simulink model "uni_model_v3"  (R2017b)
settings: Solver=FixedStepDiscrete  StartTime=0.0  StopTime=time  FixedStep=dt  RelTol=1e-3
values from neighbouring files (symbols this model uses):
  dt = 0.1    [extendedKalmanFilter.m]    (also in matlab.mat; runV3.m; rungen.m; runpathfollower.m)
  i0 = 0    [matlab.mat]    (also in runV3.m = [0 0]')
  xi0 = [0 0 0 0 0 0 0 0]    [matlab.mat]    (also in runV3.m = [0 0 0 0 0 0 0 0]'; runpathfollower.m = [xi,yi,0,0,0,0,theta_mi,0]'; runpathplanner.m = [xi,yi,0,0,0,0,theta_mi,0]')
undefined symbols (not defined in the file or in its folder): DiscIntNeverNeededParam
libraries: simulink x13
settings Model: Creator=nisha  LastModifiedBy=nisha

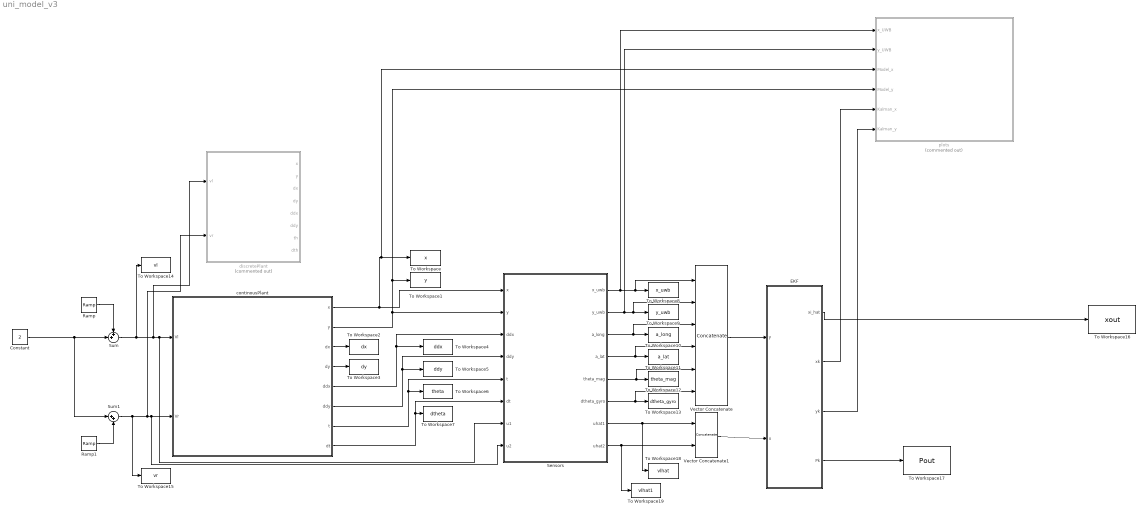
== system uni_model_v3 ==
  Constant : Constant  Value=2
  EKF : Subsystem
  Ramp : simulink/Sources/Ramp  slope=0.1  start=2  X0=0
  Ramp1 : simulink/Sources/Ramp  slope=0.1  start=3  X0=0
  Sensors : Subsystem  Description=dfg
  Sum : Sum  Inputs=++|
  Sum1 : Sum  Inputs=|++
  To Workspace : ToWorkspace  VariableName=x  SampleTime=-1
  To Workspace1 : ToWorkspace  VariableName=y  SampleTime=-1
  To Workspace10 : ToWorkspace  VariableName=a_long  SampleTime=-1
  To Workspace11 : ToWorkspace  VariableName=a_lat  SampleTime=-1
  To Workspace12 : ToWorkspace  VariableName=theta_mag  SampleTime=-1
  To Workspace13 : ToWorkspace  VariableName=dtheta_gyro  SampleTime=-1
  To Workspace14 : ToWorkspace  VariableName=vl  SampleTime=-1
  To Workspace15 : ToWorkspace  VariableName=vr  SampleTime=-1
  To Workspace16 : ToWorkspace  VariableName=xout  SampleTime=-1
  To Workspace17 : ToWorkspace  VariableName=Pout  SampleTime=-1
  To Workspace18 : ToWorkspace  VariableName=vlhat  SampleTime=-1
  To Workspace19 : ToWorkspace  VariableName=vlhat1  SampleTime=-1
  To Workspace2 : ToWorkspace  VariableName=dx  SampleTime=-1
  To Workspace3 : ToWorkspace  VariableName=dy  SampleTime=-1
  To Workspace4 : ToWorkspace  VariableName=ddx  SampleTime=-1
  To Workspace5 : ToWorkspace  VariableName=ddy  SampleTime=-1
  To Workspace6 : ToWorkspace  VariableName=theta  SampleTime=-1
  To Workspace7 : ToWorkspace  VariableName=dtheta  SampleTime=-1
  To Workspace8 : ToWorkspace  VariableName=x_uwb  SampleTime=-1
  To Workspace9 : ToWorkspace  VariableName=y_uwb  SampleTime=-1
  Vector Concatenate : Concatenate  NumInputs=6
  Vector Concatenate1 : Concatenate
  continousPlant : Subsystem  TreatAsAtomicUnit=on
  discretePlant : Subsystem  Commented=on
  plots : Subsystem  Commented=on
  wires:
  Constant/1 -> Sum1/1, Sum/2
  Sum/1 -> To Workspace14/1, discretePlant/1(vl), Sensors/7(u1), continousPlant/1(Vl)
  Ramp/1 -> Sum/1
  Ramp1/1 -> Sum1/2
  continousPlant/1(x) -> plots/3(Model_x), To Workspace/1, Sensors/1(x)
  continousPlant/2(y) -> plots/4(Model_y), To Workspace1/1, Sensors/2(y)
  continousPlant/3(dx) -> To Workspace2/1
  continousPlant/4(dy) -> To Workspace3/1
  continousPlant/5(ddx) -> Sensors/3(ddx), To Workspace4/1
  continousPlant/6(ddy) -> Sensors/4(ddy), To Workspace5/1
  continousPlant/7(t) -> Sensors/5(t), To Workspace6/1
  continousPlant/8(dt) -> Sensors/6(dt), To Workspace7/1
  Sensors/1("x_uwb ") -> plots/1(x_UWB), Vector Concatenate/1, To Workspace8/1
  Sensors/2(y_uwb) -> Vector Concatenate/2, To Workspace9/1, plots/2(y_UWB)
  Sensors/5(theta_mag) -> Vector Concatenate/5, To Workspace12/1
  Sensors/4(a_lat) -> Vector Concatenate/4, To Workspace11/1
  Sensors/6(dtheta_gyro) -> To Workspace13/1, Vector Concatenate/6
  Sensors/3(a_long) -> Vector Concatenate/3, To Workspace10/1
  Vector Concatenate/1 -> EKF/1(y)
  EKF/1(xi_hat) -> To Workspace16/1
  Vector Concatenate1/1 -> EKF/2(u)
  Sum1/1 -> To Workspace15/1, discretePlant/2(vr), Sensors/8(u2), continousPlant/2(Vr)
  Sensors/7(uhat1) -> To Workspace18/1, Vector Concatenate1/1
  Sensors/8(uhat2) -> To Workspace19/1, Vector Concatenate1/2
  EKF/2(xk) -> plots/5(Kalman_x)
  EKF/3(yk) -> plots/6(Kalman_y)
  EKF/4(Pk) -> To Workspace17/1

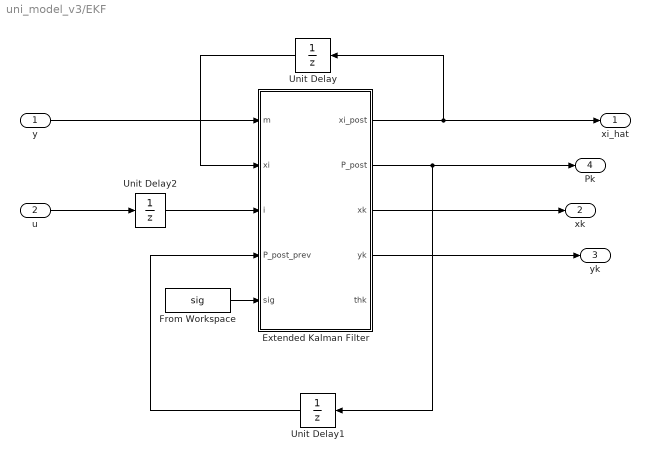
== system uni_model_v3/EKF ==
  y : Inport
  u : Inport  Port=2
  Extended Kalman Filter : MATLAB Function  TreatAsAtomicUnit=on
  From Workspace : FromWorkspace  VariableName=sig  SampleTime=0
  Unit Delay : UnitDelay  InitialCondition=xi0  SampleTime=-1
  Unit Delay1 : UnitDelay  InitialCondition=zeros(8,8)  SampleTime=-1
  Unit Delay2 : UnitDelay  InitialCondition=i0  SampleTime=-1
  xi_hat : Outport
  xk : Outport  Port=2
  yk : Outport  Port=3
  Pk : Outport  Port=4
  wires:
  Extended Kalman Filter/1(xi_post) -> xi_hat/1, Unit Delay/1
  y/1 -> Extended Kalman Filter/1(m)
  u/1 -> Unit Delay2/1
  Unit Delay2/1 -> Extended Kalman Filter/3(i)
  Unit Delay/1 -> Extended Kalman Filter/2(xi)
  Extended Kalman Filter/2(P_post) -> Unit Delay1/1, Pk/1
  Unit Delay1/1 -> Extended Kalman Filter/4(P_post_prev)
  Extended Kalman Filter/3(xk) -> xk/1
  Extended Kalman Filter/4(yk) -> yk/1
  From Workspace/1 -> Extended Kalman Filter/5(sig)

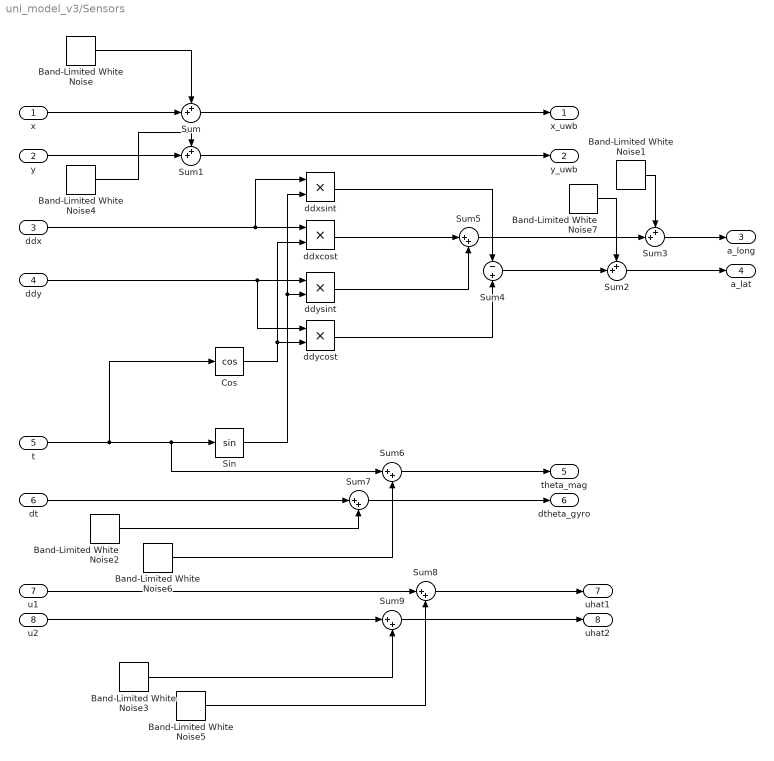
== system uni_model_v3/Sensors ==
  x : Inport
  y : Inport  Port=2
  ddx : Inport  Port=3
  ddy : Inport  Port=4
  t : Inport  Port=5
  dt : Inport  Port=6
  u1 : Inport  Port=7
  u2 : Inport  Port=8
  Band-Limited White Noise : simulink/Sources/Band-Limited White Noise  Cov=noiseUWB  Ts=dt  seed=[23341]
  Band-Limited White Noise1 : simulink/Sources/Band-Limited White Noise  Cov=noiseAcc  Ts=dt  seed=[23341]
  Band-Limited White Noise2 : simulink/Sources/Band-Limited White Noise  Cov=noiseGyro  Ts=dt  seed=[23341]
  Band-Limited White Noise3 : simulink/Sources/Band-Limited White Noise  Cov=noiseIn  Ts=dt  seed=[23341]
  Band-Limited White Noise4 : simulink/Sources/Band-Limited White Noise  Cov=noiseUWB  Ts=dt  seed=[23241]
  Band-Limited White Noise5 : simulink/Sources/Band-Limited White Noise  Cov=noiseIn  Ts=dt  seed=[23341]
  Band-Limited White Noise6 : simulink/Sources/Band-Limited White Noise  Cov=noiseMag  Ts=dt  seed=[23341]
  Band-Limited White Noise7 : simulink/Sources/Band-Limited White Noise  Cov=noiseAcc  Ts=dt  seed=[23341]
  Cos : Trigonometry  Operator=cos
  Sin : Trigonometry
  Sum{,1..3} (4 alike) : Sum  Inputs=++|
  Sum4 : Sum  Inputs=-|+
  Sum{5..9} (5 alike) : Sum  Inputs=|++
  ddxcost : Product
  ddxsint : Product
  ddycost : Product
  ddysint : Product
  "x_uwb " : Outport
  y_uwb : Outport  Port=2
  a_long : Outport  Port=3
  a_lat : Outport  Port=4
  theta_mag : Outport  Port=5
  dtheta_gyro : Outport  Port=6
  uhat1 : Outport  Port=7
  uhat2 : Outport  Port=8
  wires:
  x/1 -> Sum/2
  y/1 -> Sum1/2
  Band-Limited White Noise/1 -> Sum/1
  Sum/1 -> "x_uwb "/1
  Sum1/1 -> y_uwb/1
  Band-Limited White Noise1/1 -> Sum3/1
  t/1 -> Sum6/1, Sin/1, Cos/1
  ddx/1 -> ddxcost/1, ddxsint/1
  Cos/1 -> ddxcost/2, ddycost/2
  Sin/1 -> ddxsint/2, ddysint/2
  ddy/1 -> ddycost/1, ddysint/1
  Sum5/1 -> Sum3/2
  Sum4/1 -> Sum2/2
  ddxcost/1 -> Sum5/1
  ddysint/1 -> Sum5/2
  ddxsint/1 -> Sum4/1
  ddycost/1 -> Sum4/2
  Sum6/1 -> theta_mag/1
  dt/1 -> Sum7/1
  Sum7/1 -> dtheta_gyro/1
  Band-Limited White Noise2/1 -> Sum7/2
  Sum3/1 -> a_long/1
  Sum2/1 -> a_lat/1
  Band-Limited White Noise3/1 -> Sum9/2
  Sum9/1 -> uhat2/1
  u2/1 -> Sum9/1
  Sum8/1 -> uhat1/1
  u1/1 -> Sum8/1
  Band-Limited White Noise4/1 -> Sum1/1
  Band-Limited White Noise5/1 -> Sum8/2
  Band-Limited White Noise6/1 -> Sum6/2
  Band-Limited White Noise7/1 -> Sum2/1

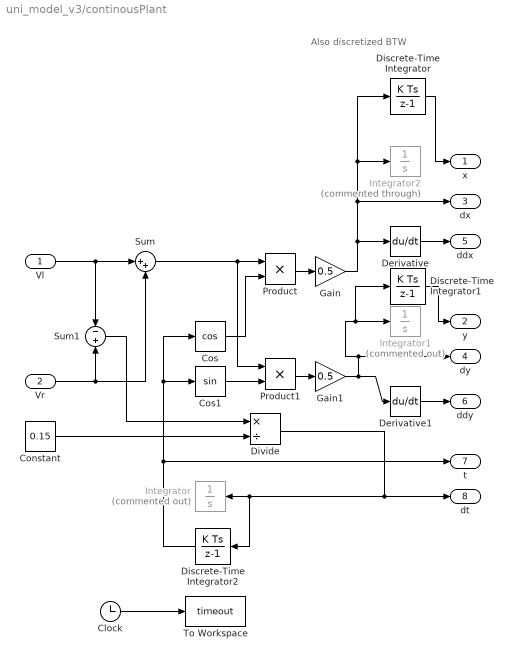
== system uni_model_v3/continousPlant ==
  note: Also discretized BTW
  Vl : Inport
  Vr : Inport  Port=2
  Clock : Clock
  Constant : Constant  Value=0.15
  Cos : Trigonometry  Operator=cos
  Cos1 : Trigonometry
  Derivative : Derivative
  Derivative1 : Derivative
  Discrete-Time Integrator : DiscreteIntegrator  InitialConditionSetting=State (most efficient)  SampleTime=-1  ICPrevOutput=DiscIntNeverNeededParam  ICPrevScaledInput=DiscIntNeverNeededParam
  Discrete-Time Integrator1 : DiscreteIntegrator  InitialConditionSetting=State (most efficient)  SampleTime=-1  ICPrevOutput=DiscIntNeverNeededParam  ICPrevScaledInput=DiscIntNeverNeededParam
  Discrete-Time Integrator2 : DiscreteIntegrator  InitialConditionSetting=State (most efficient)  SampleTime=-1  ICPrevOutput=DiscIntNeverNeededParam  ICPrevScaledInput=DiscIntNeverNeededParam
  Divide : Product  Inputs=*/
  Gain : Gain  Gain=0.5
  Gain1 : Gain  Gain=0.5
  Integrator : Integrator  Commented=on
  Integrator1 : Integrator  Commented=on
  Integrator2 : Integrator  Commented=through
  Product : Product
  Product1 : Product
  Sum : Sum  Inputs=|++
  Sum1 : Sum  Inputs=-|+
  To Workspace : ToWorkspace  VariableName=timeout  SampleTime=-1
  x : Outport
  y : Outport  Port=2
  dx : Outport  Port=3
  dy : Outport  Port=4
  ddx : Outport  Port=5
  ddy : Outport  Port=6
  t : Outport  Port=7
  dt : Outport  Port=8
  wires:
  Vl/1 -> Sum/1, Sum1/1
  Vr/1 -> Sum/2, Sum1/2
  Sum/1 -> Product1/1, Product/1
  Product1/1 -> Gain1/1
  Product/1 -> Gain/1
  Gain1/1 -> Discrete-Time Integrator1/1, Integrator1/1, dy/1, Derivative1/1
  Constant/1 -> Divide/2
  Divide/1 -> Discrete-Time Integrator2/1, Integrator/1, dt/1
  Sum1/1 -> Divide/1
  Cos/1 -> Product/2
  Cos1/1 -> Product1/2
  Discrete-Time Integrator2/1 -> t/1, Cos1/1, Cos/1
  Discrete-Time Integrator1/1 -> y/1
  Gain/1 -> Derivative/1, Discrete-Time Integrator/1, Integrator2/1, dx/1
  Clock/1 -> To Workspace/1
  Derivative/1 -> ddx/1
  Derivative1/1 -> ddy/1
  Discrete-Time Integrator/1 -> x/1

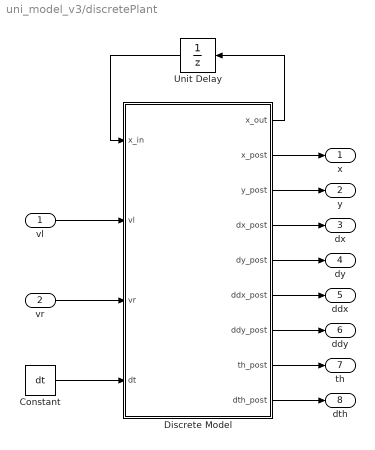
== system uni_model_v3/discretePlant ==
  vl : Inport
  vr : Inport  Port=2
  Constant : Constant  Value=dt
  Discrete Model : MATLAB Function  TreatAsAtomicUnit=on
  Unit Delay : UnitDelay  InitialCondition=xi0  SampleTime=-1
  x : Outport
  y : Outport  Port=2
  dx : Outport  Port=3
  dy : Outport  Port=4
  ddx : Outport  Port=5
  ddy : Outport  Port=6
  th : Outport  Port=7
  dth : Outport  Port=8
  wires:
  vl/1 -> Discrete Model/2(vl)
  Discrete Model/1(x_out) -> Unit Delay/1
  Unit Delay/1 -> Discrete Model/1(x_in)
  vr/1 -> Discrete Model/3(vr)
  Discrete Model/2(x_post) -> x/1
  Discrete Model/3(y_post) -> y/1
  Discrete Model/4(dx_post) -> dx/1
  Discrete Model/5(dy_post) -> dy/1
  Discrete Model/6(ddx_post) -> ddx/1
  Discrete Model/7(ddy_post) -> ddy/1
  Discrete Model/8(th_post) -> th/1
  Discrete Model/9(dth_post) -> dth/1
  Constant/1 -> Discrete Model/4(dt)

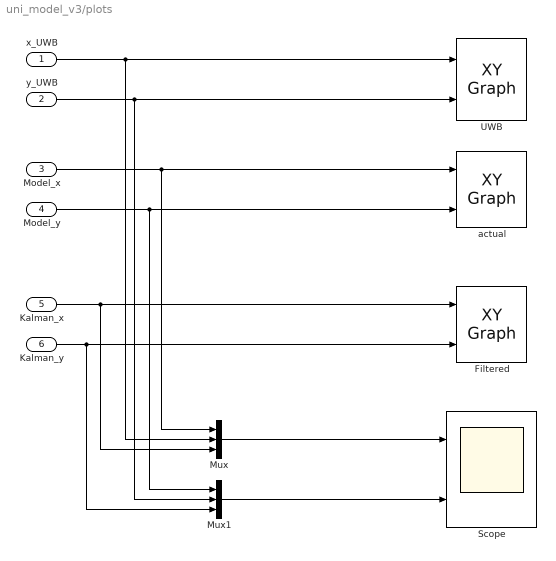
== system uni_model_v3/plots ==
  x_UWB : Inport
  y_UWB : Inport  Port=2
  Model_x : Inport  Port=3
  Model_y : Inport  Port=4
  Kalman_x : Inport  Port=5
  Kalman_y : Inport  Port=6
  Filtered : simulink/Sinks/XY Graph  xmin=-5  xmax=15  ymin=-15  ymax=10  st=-1
  Mux : Mux  Inputs=3
  Mux1 : Mux  Inputs=3
  Scope : Scope  NumInputPorts=2
  UWB : simulink/Sinks/XY Graph  xmin=-5  xmax=15  ymin=-15  ymax=10  st=-1
  actual : simulink/Sinks/XY Graph  xmin=-5  xmax=15  ymin=-15  ymax=10  st=-1
  wires:
  Mux/1 -> Scope/1
  Mux1/1 -> Scope/2
  x_UWB/1 -> Mux/2, UWB/1
  Kalman_y/1 -> Mux1/3, Filtered/2
  Model_y/1 -> Mux1/1, actual/2
  Model_x/1 -> Mux/1, actual/1
  Kalman_x/1 -> Mux/3, Filtered/1
  y_UWB/1 -> Mux1/2, UWB/2

== matlab function uni_model_v3/discretePlant/Discrete Model ==
  data: x_in input; x_out output; vl input; vr input; x_post output; y_post output; dx_post output; dy_post output; ddx_post output; ddy_post output; th_post output; dth_post output; dt input
function [x_out,x_post,y_post,dx_post,dy_post,ddx_post,ddy_post,th_post,dth_post]         = fcn(x_in,vl, vr,dt)

d=0.15;
x=x_in(1); y=x_in(2); dx=x_in(3);dy=x_in(4);ddx=x_in(5);ddy=x_in(6); phi=x_in(7); dphi=x_in(8);
th=phi+0.5*dphi*dt;
x_out = ...
[x + dx*dt + ddx*dt^2/2
 y + dy*dt + ddy*dt^2/2
 (vl+vr)/2*cos(th)+ddx*dt
 (vl+vr)/2*sin(th)+ddy*dt
 ddx
 ddy
 phi + dphi*dt
 (vr-vl)/d];

x_post=x_out(1); y_post=x_out(2); dx_post=x_out(3);dy_post=x_out(4);ddx_post=x_out(5);ddy_post=x_out(6);th_post=x_out(7);dth_post=x_out(8);
end

== matlab function uni_model_v3/EKF/Extended Kalman Filter ==
  data: m input; xi input; i input; P_post_prev input; xi_post output; P_post output; xk output; yk output; sig input; thk output
function [xi_post,P_post,xk,yk, thk] = fcn(m,xi,i,P_post_prev,sig)
%% Prediction

d=0.15; dt=0.1;
x=xi(1); y=xi(2); dx=xi(3); dy=xi(4); ddx=xi(5); ddy=xi(6); phi=xi(7); dphi=xi(8);
th=phi+0.5*dphi*dt;
vl=i(1); vr=i(2);
xi_prio = ...
            [ x + dx*dt + ddx*dt^2/2
              y + dy*dt + ddy*dt^2/2
             (vl+vr)/2*cos(th)+ddx*dt
             (vl+vr)/2*sin(th)+ddy*dt
             ddx
             ddy
             phi + dphi*dt
             (vr-vl)/d               ];

A = ...
        [ 1, 0, dt,  0, dt^2/2,      0,                              0,                             0
          0, 1,  0, dt,      0, dt^2/2,                              0,                             0
          0, 0,  0,  0,     dt,      0,         -sin(th)*(vl/2 + vr/2), -(dt*sin(th)*(vl/2 + vr/2))/2
          0, 0,  0,  0,      0,     dt,          cos(th)*(vl/2 + vr/2),  (dt*cos(th)*(vl/2 + vr/2))/2
          0, 0,  0,  0,      1,      0,                              0,                             0
          0, 0,  0,  0,      0,      1,                              0,                             0
          0, 0,  0,  0,      0,      0,                              1,                             dt
          0, 0,  0,  0,      0,      0,                              0,                             0];

V= ...
    [         0,         0
              0,         0
      cos(th)/2, cos(th)/2
      sin(th)/2, sin(th)/2
              0,         0
              0,         0
              0,         0
           -1/d,       1/d];
sigx=sig(1);sigy=sig(2);sigdx=sig(3);sigdy=sig(4);sigddx=sig(5);sigddy=sig(6);sigphi=sig(7);
sigdphi=sig(8);sigvl=sig(9);sigvr=sig(9);

Q = diag([sigx,sigy,sigdx,sigdy,sigddx,sigddy,sigphi,sigdphi]);
M=diag([sigvl,sigvr]);
P_prio = A*P_post_prev*A'+Q + V*M*V';

%% Update
zhat = [1    0   0   0   0           0           0   0
        0    1   0   0   0           0           0   0
        0    0   0   0   cos(phi)    sin(phi)    0   0
        0    0   0   0   -sin(phi)   cos(phi)    0   0
        0    0   0   0   0           0           1   0
        0    0   0   0   0           0           0   1]*xi_prio;
C =  [1, 0, 0, 0,         0,        0,                             0, 0;
      0, 1, 0, 0,         0,        0,                             0, 0;
      0, 0, 0, 0,  cos(phi), sin(phi),   ddy*cos(phi) - ddx*sin(phi), 0;
      0, 0, 0, 0, -sin(phi), cos(phi), - ddx*cos(phi) - ddy*sin(phi), 0;
      0, 0, 0, 0,         0,        0,                             1, 0;
      0, 0, 0, 0,         0,        0,                             0, 1];
R = diag([9,10, 0.01/dt, 0.01/dt, 0.001/dt, 0.001/dt]);
K = P_prio*C'/(C*P_prio*C'+R);


% Update states and covariance matrix
xi_post = xi_prio + K*(m-zhat);
P_post = (eye(size(P_prio,1))-K*C)*P_prio; %*(eye(size(P_prio,1))-K*C)'+K*R*K';
xk=xi_post(1); yk=xi_post(2); thk=xi_post(7);
